simulink model "PX21es"  (R2015b)
settings: Solver=VariableStepAuto  StartTime=0.0  StopTime=1  RelTol=1e-3
settings Model: Creator=xmax1946  LastModifiedBy=xmax1946

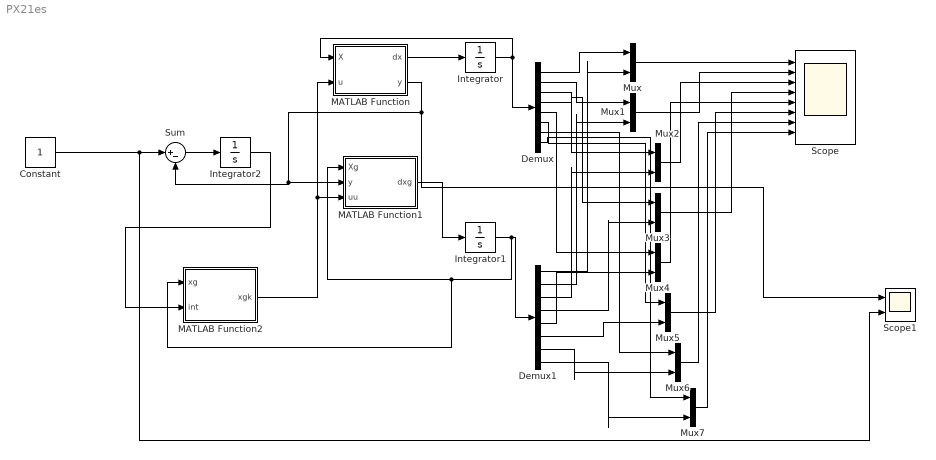
== system PX21es ==
  Constant : Constant
  Demux : Demux  Outputs=8
  Demux1 : Demux  Outputs=8
  Integrator : Integrator  InitialCondition=[0;0;0;0;0;0;0;0]
  Integrator1 : Integrator  InitialCondition=[0.05;0.05;0.05;0.05;0.05;0.05;0.05;0.05]
  Integrator2 : Integrator  IgnoreLimit=on
  MATLAB Function : MATLAB Function  TreatAsAtomicUnit=on
  MATLAB Function1 : MATLAB Function  TreatAsAtomicUnit=on
  MATLAB Function2 : MATLAB Function  TreatAsAtomicUnit=on
  Mux{,1..7} (8 alike) : Mux  Inputs=2
  Scope : Scope  NumInputPorts=8
  Scope1 : Scope  NumInputPorts=2
  Sum : Sum  Inputs=|+-
  wires:
  MATLAB Function/1(dx) -> Integrator/1
  MATLAB Function1/1(dxg) -> Integrator1/1
  Integrator/1 -> MATLAB Function/1(X), Demux/1
  MATLAB Function/2(y) -> Sum/2, MATLAB Function1/2(y), Scope1/1
  Integrator1/1 -> MATLAB Function2/1(xg), MATLAB Function1/1(Xg), Demux1/1
  Demux/1 -> Mux/1
  Demux1/1 -> Mux/2
  Demux/2 -> Mux1/1
  Demux1/2 -> Mux1/2
  Mux/1 -> Scope/1
  Mux1/1 -> Scope/2
  Constant/1 -> Scope1/2, Sum/1
  Sum/1 -> Integrator2/1
  Integrator2/1 -> MATLAB Function2/2(int)
  MATLAB Function2/1(xgk) -> MATLAB Function/2(u), MATLAB Function1/3(uu)
  Demux/3 -> Mux2/1
  Demux/4 -> Mux3/1
  Demux1/3 -> Mux2/2
  Demux1/4 -> Mux3/2
  Mux2/1 -> Scope/3
  Mux3/1 -> Scope/4
  Demux1/8 -> Mux7/2
  Demux1/7 -> Mux6/2
  Demux1/6 -> Mux5/2
  Demux1/5 -> Mux4/2
  Demux/5 -> Mux4/1
  Demux/6 -> Mux5/1
  Demux/7 -> Mux6/1
  Demux/8 -> Mux7/1
  Mux4/1 -> Scope/5
  Mux5/1 -> Scope/6
  Mux6/1 -> Scope/7
  Mux7/1 -> Scope/8

== matlab function PX21es/MATLAB Function1 ==
  data: Xg input; y input; uu input; dxg output
function dxg =fcn(Xg,y,uu)
A=[-1,2,-2,0,0,0,0,0
    0,-1,2,0,0,0,0,0
    0,-2,-1,0,0,0,0,0
    1,0,0,-2,1,0,0,0
    -1,-2,2,-1,-2,0,0,0
    0,-49,-2,0,0,-50,0,0
    0,2,-49,2,0,0,-50,2
    -1,0,-2,-48,-1,0,-2,-50];
B=[0;1;0;1;0;-1;0;-1];
C=[2,0,1,1,1,0,1,0];

% Ll=[2.7192;-.6782;.2845;-.96285;-4.4755;-1.07815;-.28459;.96285]*1e+09;
Ll=[0.01999;.49;-.02;.48;-.02999;-.4999;.0200;-.48]*1e+02;
Ll=[0.01999;1.5495;-.02;1.5395;-.02999;-1.5595;.0200;-1.5395]*1e+02;
dxg=A*Xg+B*uu+Ll*(y-C*Xg);
% [0.05;0.05;0.05;0.05;0.05;0.05;0.05;0.05]

== matlab function PX21es/MATLAB Function ==
  data: dx output; X input; y output; u input
function [dx,y]=fcn(X,u)
A=[-1,2,-2,0,0,0,0,0
    0,-1,2,0,0,0,0,0
    0,-2,-1,0,0,0,0,0
    1,0,0,-2,1,0,0,0
    -1,-2,2,-1,-2,0,0,0
    0,-49,-2,0,0,-50,0,0
    0,2,-49,2,0,0,-50,2
    -1,0,-2,-48,-1,0,-2,-50];
B=[0;1;0;1;0;-1;0;-1];
C=[2,0,1,1,1,0,1,0];

dx=A*X+B*u;
y=C*X;

== matlab function PX21es/MATLAB Function2 ==
  data: xg input; xgk output; int input
function xgk = fcn(xg,int)
kic=2.4322*1e+02;
Kc=[.3436,-1.161,2.2404,4.3906,.1718,-1.18104,2.2604,4.2388]*1e+02;

% kic=.81394*1e+02;
% Kc=[.1933,-.4713,.6972,1.54,.096,-.4913,.71727,1.4665]*1e+02;

% kic=2.503*1e+03;
% Kc=[.1979,-1.033,2.403,4.3706,.0989,-1.035,2.405,4.2736]*1e+02;
xgk=int*kic-Kc*xg;
